simulink model "Example"  (R2019b)
settings: Solver=VariableStepAuto  StartTime=0.0  StopTime=100  RelTol=1e-3
libraries: MotionSystems_Simulink x2
settings Model: EnablePacing=on  Creator=usr  LastModifiedBy=usr

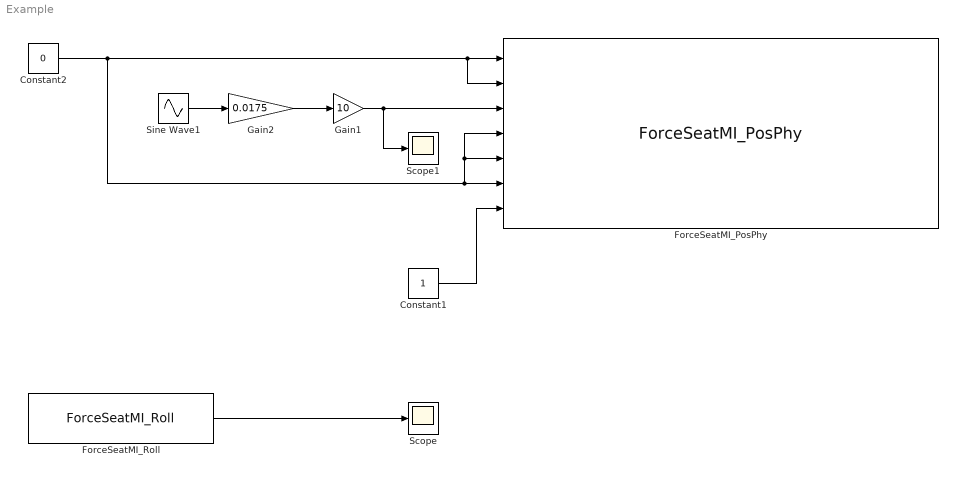
== system Example ==
  Constant1 : Constant  OutDataTypeStr=int32
  Constant2 : Constant  Value=0
  ForceSeatMI_PosPhy : MotionSystems_Simulink/ForceSeatMI_PosPhy
      settings: SourceProductName=MotionsSystems ForceSeat MI
  ForceSeatMI_Roll : MotionSystems_Simulink/ForceSeatMI_Roll
      settings: SourceProductName=MotionsSystems ForceSeatMI
  Gain1 : Gain  Gain=10
  Gain2 : Gain  Gain=0.0175
  Scope : Scope
  Scope1 : Scope
  Sine Wave1 : Sin  SampleTime=0.01
  wires:
  Constant1/1 -> ForceSeatMI_PosPhy/7
  Constant2/1 -> ForceSeatMI_PosPhy/2, ForceSeatMI_PosPhy/1, ForceSeatMI_PosPhy/4, ForceSeatMI_PosPhy/5, ForceSeatMI_PosPhy/6
  Sine Wave1/1 -> Gain2/1
  Gain2/1 -> Gain1/1
  Gain1/1 -> Scope1/1, ForceSeatMI_PosPhy/3
  ForceSeatMI_Roll/1 -> Scope/1
